simulink library "AEMACE10_INSTRUMENTATION"  (R2021b)
settings: Solver=VariableStepAuto  StartTime=0.0  StopTime=10.0  RelTol=1e-3
settings Model: Creator=ACH  LastModifiedBy=ACH

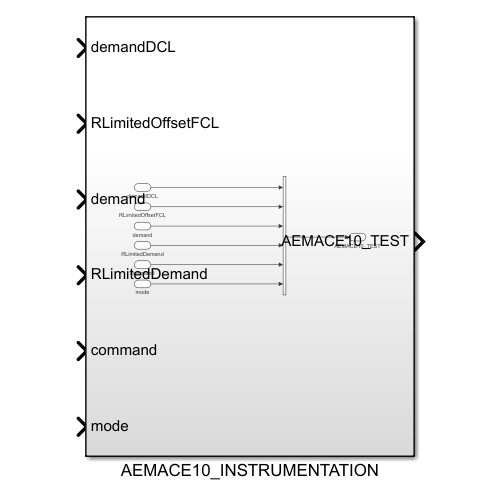
[thumbnail: Simulink's stored preview of the top-level diagram]
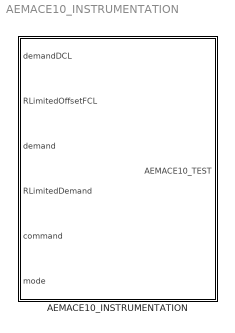
== system AEMACE10_INSTRUMENTATION ==
  AEMACE10_INSTRUMENTATION : Subsystem

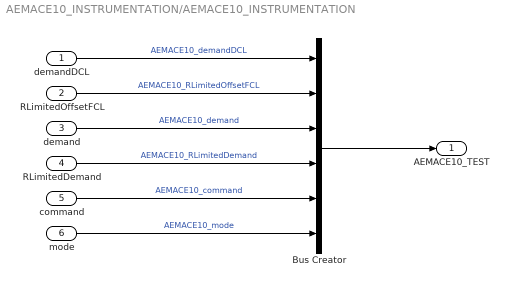
== system AEMACE10_INSTRUMENTATION/AEMACE10_INSTRUMENTATION ==
  demandDCL : Inport
  RLimitedOffsetFCL : Inport  Port=2
  demand : Inport  Port=3
  RLimitedDemand : Inport  Port=4
  command : Inport  Port=5
  mode : Inport  Port=6
  Bus Creator : BusCreator  Inputs=6  OutDataTypeStr=Bus: AEMACE10_TEST
  AEMACE10_TEST : Outport  OutDataTypeStr=Bus: AEMACE10_TEST
  wires:
  mode/1 -> Bus Creator/6  "AEMACE10_mode"
  demand/1 -> Bus Creator/3  "AEMACE10_demand"
  Bus Creator/1 -> AEMACE10_TEST/1
  command/1 -> Bus Creator/5  "AEMACE10_command"
  demandDCL/1 -> Bus Creator/1  "AEMACE10_demandDCL"
  RLimitedOffsetFCL/1 -> Bus Creator/2  "AEMACE10_RLimitedOffsetFCL"
  RLimitedDemand/1 -> Bus Creator/4  "AEMACE10_RLimitedDemand"
